simulink model "model1"  (R2020a)
settings: Solver=VariableStepAuto  StartTime=0.0  StopTime=10.0  RelTol=1e-3
model workspace (MAT data in the model file):
  F = 10
  b = 50
  k1 = 50
  k2 = 50
  m1 = 100
  m2 = 200
settings Model: Creator=PRATIKSHA  LastModifiedBy=PRATIKSHA

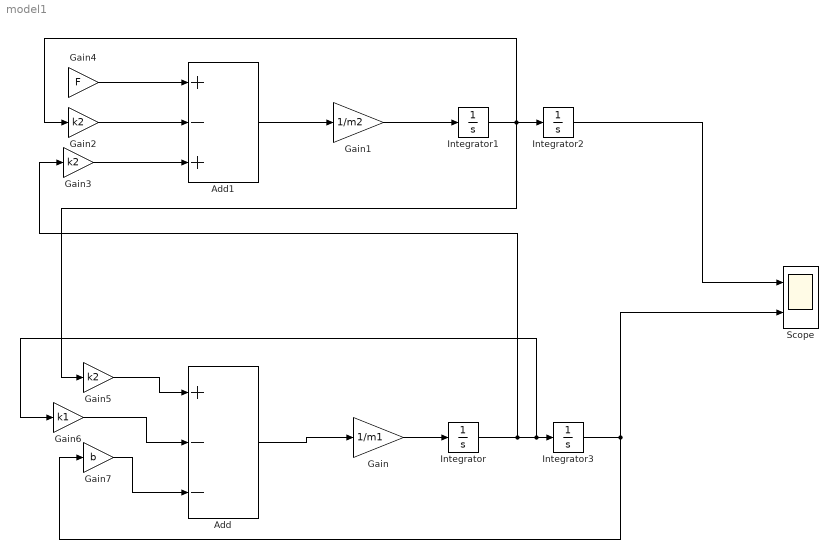
== system model1 ==
  Add : Sum  Inputs=+--
  Add1 : Sum  Inputs=+-+
  Gain : Gain  Gain=1/m1
  Gain1 : Gain  Gain=1/m2
  Gain2 : Gain  Gain=k2
  Gain3 : Gain  Gain=k2
  Gain4 : Gain  Gain=F
  Gain5 : Gain  Gain=k2
  Gain6 : Gain  Gain=k1
  Gain7 : Gain  Gain=b
  Integrator{,1..3} (4 alike) : Integrator
  Scope : Scope  NumInputPorts=2
  wires:
  Add/1 -> Gain/1
  Gain/1 -> Integrator/1
  Gain1/1 -> Integrator1/1
  Add1/1 -> Gain1/1
  Gain4/1 -> Add1/1
  Gain2/1 -> Add1/2
  Gain3/1 -> Add1/3
  Integrator2/1 -> Scope/1
  Integrator1/1 -> Gain5/1, Gain2/1, Integrator2/1
  Gain5/1 -> Add/1
  Gain6/1 -> Add/2
  Integrator/1 -> Gain6/1, Integrator3/1, Gain3/1
  Integrator3/1 -> Gain7/1, Scope/2
  Gain7/1 -> Add/3
